simulink model "Tansmissiontest"  (R2024a)
settings: Solver=ode45  StartTime=0.0  StopTime=50  RelTol=1e-3  EnableMultiTasking=on
undefined symbols (not defined in the file): alpha, alpha1, beta, beta1, c, c1, d, gamma, gamma1, k, k1, n, sigma, sigma1
libraries: fl_lib x19, nesl_utility x17, sdl_lib x7, simulink x2
settings Model: Creator=dell  LastModifiedBy=18311
settings SolverCC: AlgebraicLoopSolver=TrustRegion
settings DataIOCC: SaveFormat=StructureWithTime  ReturnWorkspaceOutputs=off
settings OptimizationCC: LifeSpan=inf
settings DebuggingCC: UnconnectedInputMsg=warning  UnconnectedOutputMsg=warning  UnconnectedLineMsg=warning  SFUnexpectedBacktrackingDiag=warning  SFNoUnconditionalDefaultTransitionDiag=warning  SFExecutionAtInitializationDiag=none  ArithmeticOperatorsInVariantConditions=warning
settings HardwareCC: ProdBitPerSizeT=32  ProdBitPerPtrDiffT=32  ProdWordSize=32  ProdHWDeviceType=Specified
settings ModelReferenceCC: EnableRefExpFcnMdlSchedulingChecks=on
settings SFSimCC: SimUseLocalCustomCode=off  CustomCodeUndefinedFunction=UseInterfaceOnly
settings RTWCC: RTWUseLocalCustomCode=off  GPUComputeCapability=3.5  DLArmComputeVersion=19.05
settings CodeAppCC: StateflowObjectComments=on
settings GRTTargetCC: TargetLangStandard=C89/C90 (ANSI)
settings ConfigComp: CovMetricSettings=dw  CovSaveCumulativeToWorkspaceVar=on  CovSaveSingleToWorkspaceVar=on  CovExternalEMLEnable=off
settings SimscapeCC: SimscapeNormalizeSystem=off

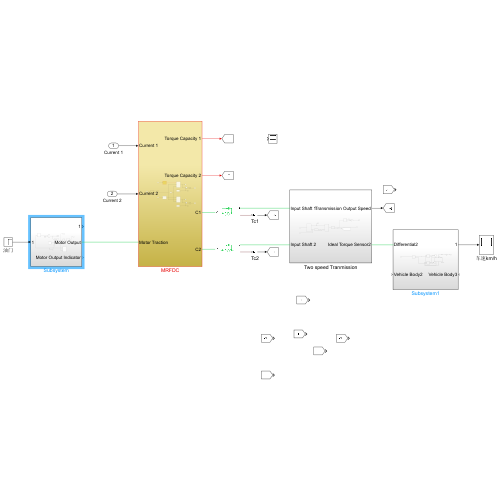
[thumbnail: Simulink's stored preview of the top-level diagram]
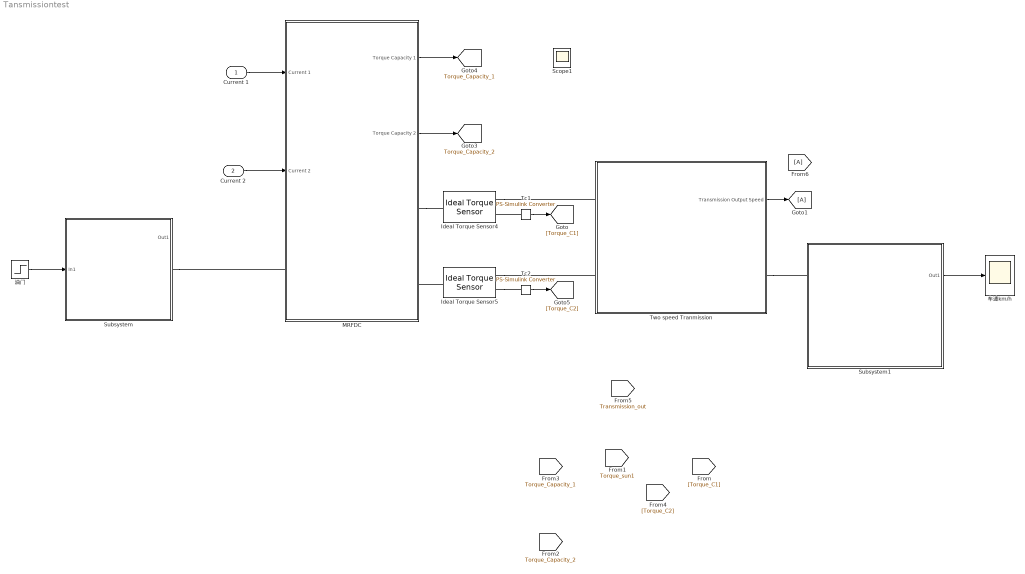
== system Tansmissiontest ==
  Current 1 : Inport
  Current 2 : Inport  Port=2
  From6 : From
  Goto1 : Goto
  Ideal Torque Sensor4 : fl_lib/Mechanical/Mechanical Sensors/Ideal Torque Sensor
  Ideal Torque Sensor5 : fl_lib/Mechanical/Mechanical Sensors/Ideal Torque Sensor
  MRFDC : Subsystem
  Scope1 : Scope
  Subsystem : Subsystem
  Subsystem1 : Subsystem
  Tc1 : nesl_utility/PS-Simulink Converter  PhysicalDomain=network_engine_domain  SubClassName=ps_output  LeftPortType=input  RightPortType=output  PseudoPeriodic=off  Frequencies=[]  VectorFormat=1-D array  Unit=1  AffineConversion=off
  Tc2 : nesl_utility/PS-Simulink Converter  PhysicalDomain=network_engine_domain  SubClassName=ps_output  LeftPortType=input  RightPortType=output  PseudoPeriodic=off  Frequencies=[]  VectorFormat=1-D array  Unit=1  AffineConversion=off
  Two speed Tranmission : Subsystem
  油门 : Step  SampleTime=0
  车速km/h : Scope
  tag scope: Torque_Capacity_1=global, Torque_Capacity_2=global
  wires:
  油门/1 -> Subsystem/1(In1)
  Current 2/1 -> MRFDC/2(Current 2)
  Current 1/1 -> MRFDC/1(Current 1)
  Tc1/1 -> [Torque_C1]
  Tc2/1 -> [Torque_C2]
  MRFDC/1(Torque Capacity 1) -> [Torque_Capacity_1]
  MRFDC/2(Torque Capacity 2) -> [Torque_Capacity_2]
  Subsystem1/1(Out1) -> 车速km/h/1
  Two speed Tranmission/1(Transmission Output Speed) -> Goto1/1
  connections:
  Subsystem/RConn1 -- MRFDC/LConn1
  Ideal Torque Sensor5/LConn1 -- MRFDC/RConn2
  MRFDC/RConn1 -- Ideal Torque Sensor4/LConn1
  Tc1/LConn1 -- Ideal Torque Sensor4/RConn2
  Ideal Torque Sensor5/RConn2 -- Tc2/LConn1
  Ideal Torque Sensor4/RConn1 -- Two speed Tranmission/LConn1
  Ideal Torque Sensor5/RConn1 -- Two speed Tranmission/LConn2
  Two speed Tranmission/RConn1 -- Subsystem1/LConn1

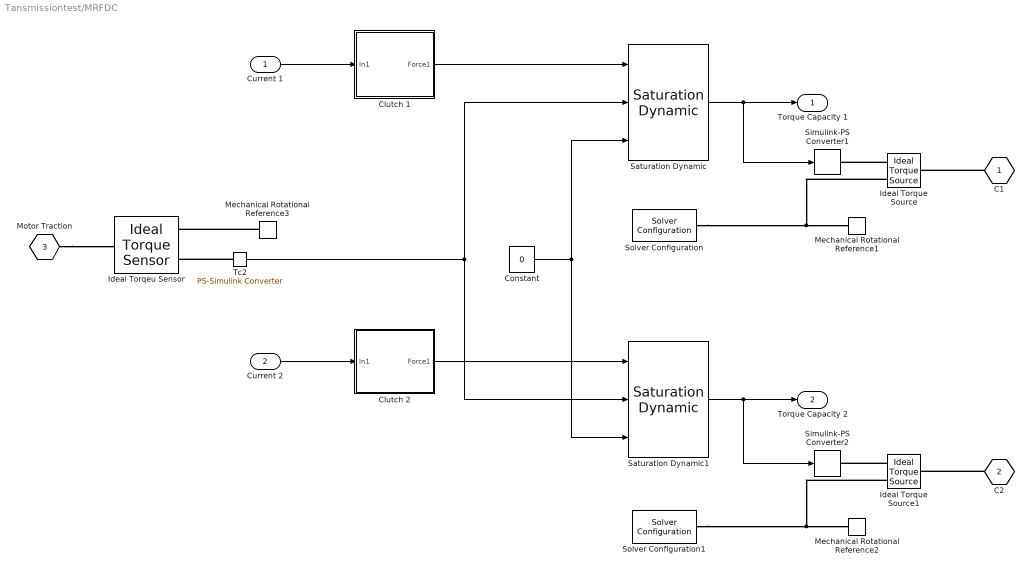
== system Tansmissiontest/MRFDC ==
  Current 1 : Inport
  Current 2 : Inport  Port=2
  Clutch 1 : Subsystem
  Clutch 2 : Subsystem
  Constant : Constant  Value=0
  Ideal Torqeu Sensor : fl_lib/Mechanical/Mechanical Sensors/Ideal Torque Sensor
  Ideal Torque Source : fl_lib/Mechanical/Mechanical Sources/Ideal Torque Source
  Ideal Torque Source1 : fl_lib/Mechanical/Mechanical Sources/Ideal Torque Source
  Mechanical Rotational Reference1 : fl_lib/Mechanical/Rotational Elements/Mechanical Rotational Reference
  Mechanical Rotational Reference2 : fl_lib/Mechanical/Rotational Elements/Mechanical Rotational Reference
  Mechanical Rotational Reference3 : fl_lib/Mechanical/Rotational Elements/Mechanical Rotational Reference
  Saturation Dynamic : simulink/Discontinuities/Saturation Dynamic  OutMin=[]  OutMax=[]  OutDataTypeStr=Inherit: Same as second input  OutDataType=fixdt(1, 16)  OutScaling=2^-10  DoSatur=off
  Saturation Dynamic1 : simulink/Discontinuities/Saturation Dynamic  OutMin=[]  OutMax=[]  OutDataTypeStr=Inherit: Same as second input  OutDataType=fixdt(1, 16)  OutScaling=2^-10  DoSatur=off
  Simulink-PS Converter1 : nesl_utility/Simulink-PS Converter  PhysicalDomain=network_engine_domain  SubClassName=ps_input  LeftPortType=input  RightPortType=output  PseudoPeriodic=off  Frequencies=[]  NoiseDistribution=none  NoiseParameters=[]  Unit=1  AffineConversion=off  FilteringAndDerivatives=zero  SimscapeFilterOrder=1  InputFilterTimeConstant=0.001  UdotUserProvided=1
  Simulink-PS Converter2 : nesl_utility/Simulink-PS Converter  PhysicalDomain=network_engine_domain  SubClassName=ps_input  LeftPortType=input  RightPortType=output  PseudoPeriodic=off  Frequencies=[]  NoiseDistribution=none  NoiseParameters=[]  Unit=1  AffineConversion=off  FilteringAndDerivatives=zero  SimscapeFilterOrder=1  InputFilterTimeConstant=0.001  UdotUserProvided=1
  Solver Configuration : nesl_utility/Solver Configuration  PhysicalDomain=network_engine_domain  SubClassName=solver  LeftPortType=input  RightPortType=generic  Tones=[]  Harmonics=[]  SimulateNoise=off  Profile=off  UseLocalSampling=off  EnableSwitchedLinearOptims=on  FrequencyDomain=off  UseCCode=off  RelTol=0.001  AbsTol=1e-06  MinStep=1e-09  ToWorkspace=off  RevertToSquareIcSolve=off  NumHomotopyIterations=100  PhasorMode=off  PhasorModeNumHarmonics=1  ConsistencySolver=NEWTON_FTOL  IndexReductionMethod=DerivativeReplacement  DoDC=off  ResidualTolerance=1e-09  ConsistencyTolSource=GLOBAL  ConsistencyAbsTol=0.001  ConsistencyRelTol=0.001  ConsistencyTolFactor=0.001  UseLocalSolver=on  LocalSolverChoice=NE_BACKWARD_EULER_ADVANCER  ResolveIndetEquations=on  FunctionEvalNumThread=1  LocalSolverSampleTime=0.001  DoFixedCost=on  MaxNonlinIter=3  MaxModeIter=2  ComputeImpulses=off  ImpulseIterations=2  LinearAlgebra=Sparse  LinearAlgebraNumThread=0  EquationFormulation=NE_TIME_EF  DelaysMemoryBudget=1024  AutomaticFiltering=on  FilteringTimeConstant=0.001  PartitionStorageMethod=AS_NEEDED  PartitionMemoryBudget=1024  PartitionMethod=FAST  MultibodyUseLocalSolver=off  MultibodyLocalSolverChoice=ODE1  MultibodyLocalSolverSampleTime=0.001
  Solver Configuration1 : nesl_utility/Solver Configuration  PhysicalDomain=network_engine_domain  SubClassName=solver  LeftPortType=input  RightPortType=generic  Tones=[]  Harmonics=[]  SimulateNoise=off  Profile=off  UseLocalSampling=off  EnableSwitchedLinearOptims=on  FrequencyDomain=off  UseCCode=off  RelTol=0.001  AbsTol=1e-06  MinStep=1e-09  ToWorkspace=off  RevertToSquareIcSolve=off  NumHomotopyIterations=100  PhasorMode=off  PhasorModeNumHarmonics=1  ConsistencySolver=NEWTON_FTOL  IndexReductionMethod=DerivativeReplacement  DoDC=off  ResidualTolerance=1e-09  ConsistencyTolSource=GLOBAL  ConsistencyAbsTol=0.001  ConsistencyRelTol=0.001  ConsistencyTolFactor=0.001  UseLocalSolver=on  LocalSolverChoice=NE_BACKWARD_EULER_ADVANCER  ResolveIndetEquations=on  FunctionEvalNumThread=1  LocalSolverSampleTime=0.001  DoFixedCost=on  MaxNonlinIter=3  MaxModeIter=2  ComputeImpulses=off  ImpulseIterations=2  LinearAlgebra=Sparse  LinearAlgebraNumThread=0  EquationFormulation=NE_TIME_EF  DelaysMemoryBudget=1024  AutomaticFiltering=on  FilteringTimeConstant=0.001  PartitionStorageMethod=AS_NEEDED  PartitionMemoryBudget=1024  PartitionMethod=FAST  MultibodyUseLocalSolver=off  MultibodyLocalSolverChoice=ODE1  MultibodyLocalSolverSampleTime=0.001
  Tc2 : nesl_utility/PS-Simulink Converter  PhysicalDomain=network_engine_domain  SubClassName=ps_output  LeftPortType=input  RightPortType=output  PseudoPeriodic=off  Frequencies=[]  VectorFormat=1-D array  Unit=1  AffineConversion=off
  C1 : PMIOPort  Side=Right
  C2 : PMIOPort  Port=2  Side=Right
  Motor Traction : PMIOPort  Port=3  Side=Left
  Torque Capacity 1 : Outport
  Torque Capacity 2 : Outport  Port=2
  wires:
  Current 1/1 -> Clutch 1/1(In1)
  Current 2/1 -> Clutch 2/1(In1)
  Clutch 1/1("  Force1") -> Saturation Dynamic/1
  Clutch 2/1("  Force1") -> Saturation Dynamic1/1
  Constant/1 -> Saturation Dynamic/3, Saturation Dynamic1/3
  Saturation Dynamic/1 -> Simulink-PS Converter1/1, Torque Capacity 1/1
  Saturation Dynamic1/1 -> Simulink-PS Converter2/1, Torque Capacity 2/1
  Tc2/1 -> Saturation Dynamic1/2, Saturation Dynamic/2
  connections:
  Ideal Torque Source/RConn1 -- Simulink-PS Converter1/RConn1
  Ideal Torque Source/RConn2 -- Solver Configuration/RConn1 -- Mechanical Rotational Reference1/LConn1
  Ideal Torque Source1/RConn2 -- Solver Configuration1/RConn1 -- Mechanical Rotational Reference2/LConn1
  Ideal Torque Source1/RConn1 -- Simulink-PS Converter2/RConn1
  C1/RConn1 -- Ideal Torque Source/LConn1
  C2/RConn1 -- Ideal Torque Source1/LConn1
  Motor Traction/RConn1 -- Ideal Torqeu Sensor/LConn1
  Tc2/LConn1 -- Ideal Torqeu Sensor/RConn2
  Mechanical Rotational Reference3/LConn1 -- Ideal Torqeu Sensor/RConn1

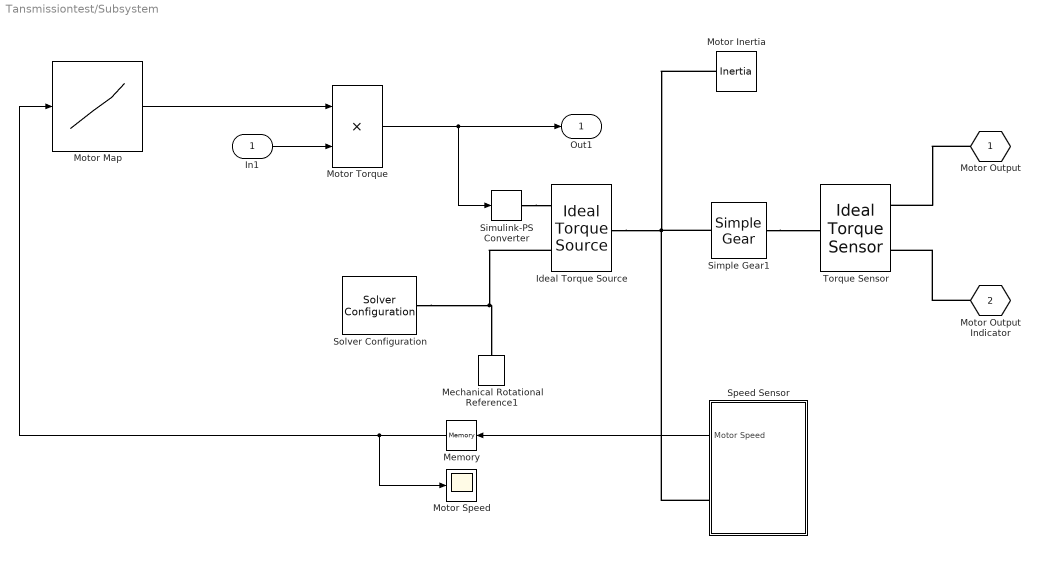
== system Tansmissiontest/Subsystem ==
  In1 : Inport
  Ideal Torque Source : fl_lib/Mechanical/Mechanical Sources/Ideal Torque Source
  Mechanical Rotational Reference1 : fl_lib/Mechanical/Rotational Elements/Mechanical Rotational Reference
  Memory : Memory
  Motor Inertia : fl_lib/Mechanical/Rotational Elements/Inertia  inertia=1 kg*m^2  num_ports=foundation.enum.numPorts2.one  w_specify=off  w_priority=High  w=0 rad/s  w_nominal_specify=off  w_nominal_value=1  w_nominal_unit=rad/s  t_specify=off  t_priority=High  t=0 N*m  t_nominal_specify=off  t_nominal_value=1  t_nominal_unit=N*m
  Motor Map : Lookup_n-D  NumberOfTableDimensions=1  BreakpointsForDimension1="[0 1000 2000 3000 4000 5000 6000 7000  7500]"  Table="[382 382.0000  382.0000  254.6667  191.0000  152.8000  127.3333  109.1429  0]"  InternalRulePriority=Speed  RndMeth=Simplest
  Motor Speed : Scope
  Motor Torque : Product
  Simple Gear1 : sdl_lib/Gears/Simple Gear  ratio=1.6  rotation_direction=3-2*(1)  enable_faults=simscape.enum.onoff.off  efficiency_fault=0.05  fault_angles=pi / 12 rad  friction_model=1  T_noload=0.1 N*m  T_nom=5 N*m  efficiency_nom=0.8  efficiency=0.8  temperature_TLU=[280, 300, 320] K  load_TLU=[1, 5, 10] N*m  efficiency_TLU=[.95, .9, .85]  efficiency_TLU2=[.85, .8, .75; .95, .9, .85; .85, .8, .7]  w_thr=0.01 rad/s  pwr_thr=0.001 W  enable_backlash=false  hardstop_model=simscape.enum.hardstop.smooth  backlash_distance=1e-3 mm  r_base=0.1 m  transition=1e-4 mm  backlash_stiffness=1e7 N/m  backlash_damping=1e6 N*s/m  coeff_rest=0  v_tol=0.001 m/s  f_tol=0 N  mu_visc=[ 0 0 ] N*m/(rad/s)  thermal_mass=50 J/K  temperature_specify=off  temperature_priority=High  temperature=300 K  temperature_nominal_specify=off  temperature_nominal_value=1  temperature_nominal_unit=K  x_backlash_specify=off  x_backlash_priority=None  x_backlash=0 mm  x_backlash_nominal_specify=off  x_backlash_nominal_value=1  x_backlash_nominal_unit=mm  f_hardstop_specify=off  f_hardstop_priority=None  f_hardstop=0 N  f_hardstop_nominal_specify=off  f_hardstop_nominal_value=1  f_hardstop_nominal_unit=N  v_backlash_specify=off  v_backlash_priority=None  v_backlash=0 m/s  v_backlash_nominal_specify=off  v_backlash_nominal_value=1  v_backlash_nominal_unit=m/s
  Simulink-PS Converter : nesl_utility/Simulink-PS Converter  PhysicalDomain=network_engine_domain  SubClassName=ps_input  LeftPortType=input  RightPortType=output  PseudoPeriodic=off  Frequencies=[]  NoiseDistribution=none  NoiseParameters=[]  Unit=1  AffineConversion=off  FilteringAndDerivatives=zero  SimscapeFilterOrder=1  InputFilterTimeConstant=0.001  UdotUserProvided=1
  Solver Configuration : nesl_utility/Solver Configuration  PhysicalDomain=network_engine_domain  SubClassName=solver  LeftPortType=input  RightPortType=generic  Tones=[]  Harmonics=[]  SimulateNoise=off  Profile=off  UseLocalSampling=off  EnableSwitchedLinearOptims=on  FrequencyDomain=off  UseCCode=off  RelTol=0.001  AbsTol=1e-06  MinStep=1e-09  ToWorkspace=off  RevertToSquareIcSolve=off  NumHomotopyIterations=100  PhasorMode=off  PhasorModeNumHarmonics=1  ConsistencySolver=NEWTON_FTOL  IndexReductionMethod=DerivativeReplacement  DoDC=off  ResidualTolerance=1e-09  ConsistencyTolSource=GLOBAL  ConsistencyAbsTol=0.001  ConsistencyRelTol=0.001  ConsistencyTolFactor=0.001  UseLocalSolver=on  LocalSolverChoice=NE_BACKWARD_EULER_ADVANCER  ResolveIndetEquations=on  FunctionEvalNumThread=1  LocalSolverSampleTime=0.001  DoFixedCost=on  MaxNonlinIter=3  MaxModeIter=2  ComputeImpulses=off  ImpulseIterations=2  LinearAlgebra=Sparse  LinearAlgebraNumThread=0  EquationFormulation=NE_TIME_EF  DelaysMemoryBudget=1024  AutomaticFiltering=on  FilteringTimeConstant=0.001  PartitionStorageMethod=AS_NEEDED  PartitionMemoryBudget=1024  PartitionMethod=FAST  MultibodyUseLocalSolver=off  MultibodyLocalSolverChoice=ODE1  MultibodyLocalSolverSampleTime=0.001
  Speed Sensor : Subsystem
  Torque Sensor : fl_lib/Mechanical/Mechanical Sensors/Ideal Torque Sensor
  Motor Output : PMIOPort  Side=Right
  Motor Output Indicator : PMIOPort  Port=2  Side=Right
  Out1 : Outport
  wires:
  Speed Sensor/1(Motor Speed) -> Memory/1
  Motor Torque/1 -> Simulink-PS Converter/1, Out1/1
  Memory/1 -> Motor Map/1, Motor Speed/1
  Motor Map/1 -> Motor Torque/1
  In1/1 -> Motor Torque/2
  connections:
  Ideal Torque Source/RConn2 -- Solver Configuration/RConn1 -- Mechanical Rotational Reference1/LConn1
  Simulink-PS Converter/RConn1 -- Ideal Torque Source/RConn1
  Ideal Torque Source/LConn1 -- Speed Sensor/RConn1 -- Simple Gear1/LConn1 -- Motor Inertia/LConn1
  Simple Gear1/RConn1 -- Torque Sensor/LConn1
  Motor Output/RConn1 -- Torque Sensor/RConn1
  Motor Output Indicator/RConn1 -- Torque Sensor/RConn2

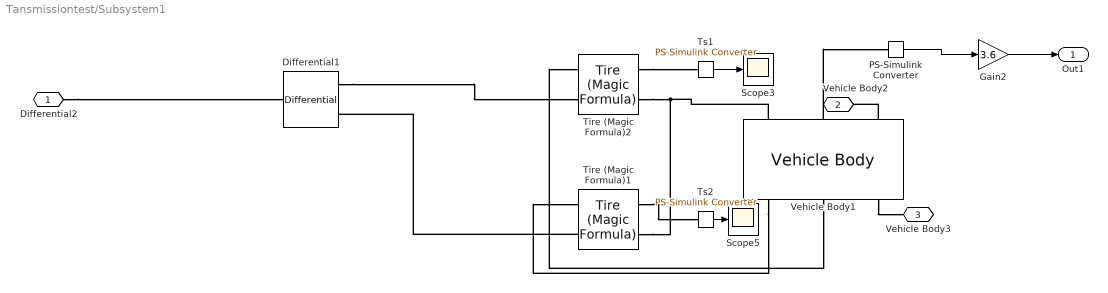
== system Tansmissiontest/Subsystem1 ==
  Differential1 : sdl_lib/Gears/Differential  driveshaft_location=2  cd_ratio=1  friction_model=1  efficiency=[ 0.85 0.92 ]  temperature_TLU=[280, 300, 320] K  efficiency_ss_TLU=[.95, .9, .85]  efficiency_cd_TLU=[.95, .9, .85]  pwr_thr=[.001, .001] W  mu_visc=[ 0 0 ] N*m/(rad/s)  model_inertia=simscape.enum.onoff.off  carrier_inertia=0.001 kg*m^2  planet_inertia=0.001 kg*m^2  thermal_mass=50 J/K  T_init=300 K
  Gain2 : Gain  Gain=3.6
  PS-Simulink Converter : nesl_utility/PS-Simulink Converter  PhysicalDomain=network_engine_domain  SubClassName=ps_output  LeftPortType=input  RightPortType=output  PseudoPeriodic=off  Frequencies=[]  VectorFormat=1-D array  Unit=1  AffineConversion=off
  Scope3 : Scope
  Scope5 : Scope
  Tire (Magic Formula)1 : sdl_lib/Tires & Vehicles/Tire (Magic Formula)  parameterization=1  F_z1=3e+3 N  F_x1=3.5e+3 N  kappa1=10  B_m=10  C_m=1.9  D_m=1  E_m=0.97  fz0=4e+3 N  p_Cx=1.685  p_Dx=[ 1.21 -0.037 ]  p_Ex=[ 0.344 0.095 -0.02 0 ]  p_Kx=[ 21.51 -0.163 0.245 ]  p_Hx=[ -0.002 0.002 ]  p_Vx=[ 0 0 ]  rolling_radius_model=sdl.enum.RollingRadiusParameterization.Constant  r_e=0.3 m  r_0=0.3 m  breff=8.39  dreff=0.26  freff=0.074  q_re0=0.99  q_v1=0.008  longvl=17 m/s  cz=5e5 N/m  model_resistance=1  resistance_model=1  coeff=0.015  p_tire=250e3 Pa  alpha=-0.003  beta=0.97  coeff_a=84e-4  coeff_b=6.2e-4 s/m  coeff_c=1.6e-4 s^2/m^2  p_tire0=240e3 Pa  fz0_resistance=4000 N  vH0=16 m/s  q_Sy=[.0082, 0, .0014, .001, 0, 0, 1.08, -.5]  v_thr=1e-3 m/s  enable_scaling_coefficients=false  lfzO=1  lcx=1  lmux=1  lex=1  lkx=1  lhx=1  lvx=1  lmy=1  model_compliance=0  stiffness=1e+6 N/m  damping=1000 N/(m/s)  model_inertia=1  inertia=1 kg*m^2  initial_velocity=0 rad/s  vxlow=0.1 m/s  v_tr_thr=0.1*(0.1) m/s  kpumin=-1e5  kpumax=1e5
  Tire (Magic Formula)2 : sdl_lib/Tires & Vehicles/Tire (Magic Formula)  parameterization=1  F_z1=3e+3 N  F_x1=3.5e+3 N  kappa1=10  B_m=10  C_m=1.9  D_m=1  E_m=0.97  fz0=4e+3 N  p_Cx=1.685  p_Dx=[ 1.21 -0.037 ]  p_Ex=[ 0.344 0.095 -0.02 0 ]  p_Kx=[ 21.51 -0.163 0.245 ]  p_Hx=[ -0.002 0.002 ]  p_Vx=[ 0 0 ]  rolling_radius_model=sdl.enum.RollingRadiusParameterization.Constant  r_e=0.3 m  r_0=0.3 m  breff=8.39  dreff=0.26  freff=0.074  q_re0=0.99  q_v1=0.008  longvl=17 m/s  cz=5e5 N/m  model_resistance=1  resistance_model=1  coeff=0.015  p_tire=250e3 Pa  alpha=-0.003  beta=0.97  coeff_a=84e-4  coeff_b=6.2e-4 s/m  coeff_c=1.6e-4 s^2/m^2  p_tire0=240e3 Pa  fz0_resistance=4000 N  vH0=16 m/s  q_Sy=[.0082, 0, .0014, .001, 0, 0, 1.08, -.5]  v_thr=1e-3 m/s  enable_scaling_coefficients=false  lfzO=1  lcx=1  lmux=1  lex=1  lkx=1  lhx=1  lvx=1  lmy=1  model_compliance=0  stiffness=1e+6 N/m  damping=1000 N/(m/s)  model_inertia=1  inertia=1 kg*m^2  initial_velocity=0 rad/s  vxlow=0.1 m/s  v_tr_thr=0.1*(0.1) m/s  kpumin=-1e5  kpumax=1e5
  Ts1 : nesl_utility/PS-Simulink Converter  PhysicalDomain=network_engine_domain  SubClassName=ps_output  LeftPortType=input  RightPortType=output  PseudoPeriodic=off  Frequencies=[]  VectorFormat=1-D array  Unit=1  AffineConversion=off
  Ts2 : nesl_utility/PS-Simulink Converter  PhysicalDomain=network_engine_domain  SubClassName=ps_output  LeftPortType=input  RightPortType=output  PseudoPeriodic=off  Frequencies=[]  VectorFormat=1-D array  Unit=1  AffineConversion=off
  Vehicle Body1 : sdl_lib/Tires & Vehicles/Vehicle Body  mass=1500 kg  n_w=2  x_f=1.4 m  x_r=1.6 m  y_c=0.5 m  mass_var=simscape.enum.onoff.off  g=9.81 m/s^2  liftoff_warning=simscape.enum.onoff.off  area=3 m^2  Cd=0.4  rho=1.18 kg/m^3  model_pitch=simscape.enum.onoff.off  inertia=4000 kg*m^2  suspension_model=sdl.enum.linearTLU.linear  k_f=1e4 N/m  b_f=1e4 N/(m/s)  k_r=1e4 N/m  b_r=1e4 N/(m/s)  k_f_TLU=[-2000, -1000, 0, 1000, 2000] N  x_f_TLU=[-.4, -.2, 0, .2, .4] m  b_f_TLU=[-200, -100, 0, 100, 200] N  v_f_TLU=[-4, -2, 0, 2, 4] m/s  k_r_TLU=[-2000, -1000, 0, 1000, 2000] N  x_r_TLU=[-.4, -.2, 0, .2, .4] m  b_r_TLU=[-200, -100, 0, 100, 200] N  v_r_TLU=[-4, -2, 0, 2, 4] m/s  interp_method=simscape.enum.interpolation.linear  extrap_method=simscape.enum.extrapolation.linear  model_hardstop=simscape.enum.onoff.off  upper_bound_f=.25 m  lower_bound_f=-.25 m  stop_k_f=1e6 N/m  stop_b_f=150 N/(m/s)  upper_bound_r=.25 m  lower_bound_r=-.25 m  stop_k_r=1e6 N/m  stop_b_r=150 N/(m/s)  initial_pitch=0 rad  initial_pitch_rate=0 rad/s  v_specify=on  v_priority=High  v=0 m/s  v_nominal_specify=off  v_nominal_value=1  v_nominal_unit=m/s
  Differential2 : PMIOPort  Side=Left
  Vehicle Body2 : PMIOPort  Port=2  Side=Left
  Vehicle Body3 : PMIOPort  Port=3  Side=Right
  Out1 : Outport
  wires:
  Ts2/1 -> Scope5/1
  Gain2/1 -> Out1/1
  PS-Simulink Converter/1 -> Gain2/1
  Ts1/1 -> Scope3/1
  connections:
  Tire (Magic Formula)1/RConn1 -- Ts2/LConn1
  Differential1/RConn2 -- Tire (Magic Formula)2/LConn2
  Vehicle Body1/LConn2 -- PS-Simulink Converter/LConn1
  Vehicle Body1/RConn2 -- Tire (Magic Formula)2/LConn1
  Vehicle Body1/RConn1 -- Tire (Magic Formula)1/LConn1
  Tire (Magic Formula)1/LConn2 -- Differential1/RConn1
  Tire (Magic Formula)2/RConn1 -- Ts1/LConn1
  Tire (Magic Formula)1/RConn2 -- Vehicle Body1/LConn1 -- Tire (Magic Formula)2/RConn2
  Vehicle Body1/RConn3 -- Vehicle Body3/RConn1
  Differential2/RConn1 -- Differential1/LConn1
  Vehicle Body1/LConn3 -- Vehicle Body2/RConn1

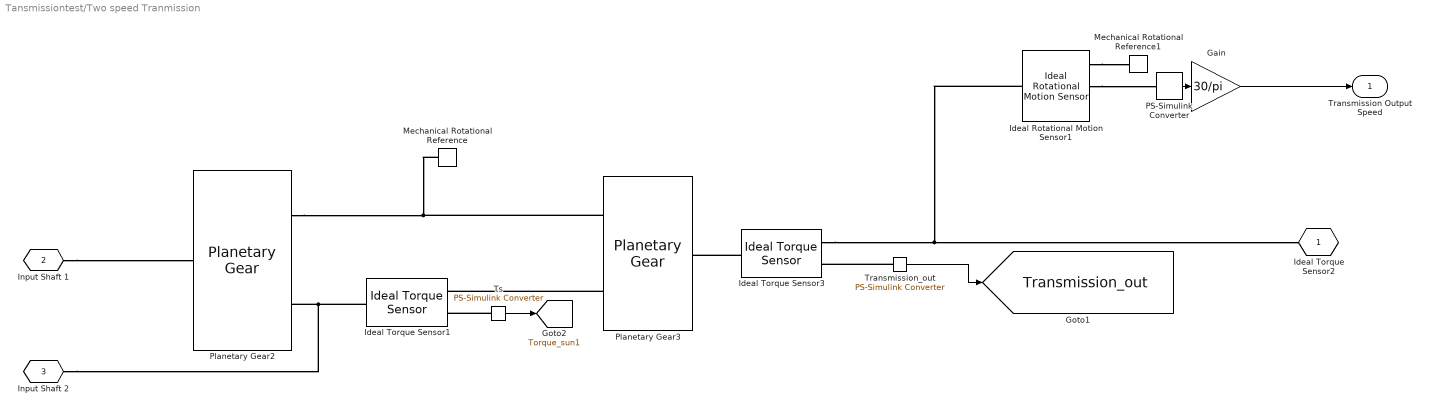
== system Tansmissiontest/Two speed Tranmission ==
  Gain : Gain  Gain=30/pi
  Ideal Rotational Motion Sensor1 : fl_lib/Mechanical/Mechanical Sensors/Ideal Rotational Motion Sensor  reference=foundation.enum.MeasurementReference.difference  acceleration_port=false  velocity_port=true  position_port=true  wrap_angle=simscape.enum.onoff.off  offset=0 rad
  Ideal Torque Sensor1 : fl_lib/Mechanical/Mechanical Sensors/Ideal Torque Sensor
  Ideal Torque Sensor3 : fl_lib/Mechanical/Mechanical Sensors/Ideal Torque Sensor
  Mechanical Rotational Reference : fl_lib/Mechanical/Rotational Elements/Mechanical Rotational Reference
  Mechanical Rotational Reference1 : fl_lib/Mechanical/Rotational Elements/Mechanical Rotational Reference
  PS-Simulink Converter : nesl_utility/PS-Simulink Converter  PhysicalDomain=network_engine_domain  SubClassName=ps_output  LeftPortType=input  RightPortType=output  PseudoPeriodic=off  Frequencies=[]  VectorFormat=1-D array  Unit=1  AffineConversion=off
  Planetary Gear2 : sdl_lib/Gears/Planetary Gear  rs_ratio=1.5  friction_model=1  efficiency=[ 0.96 0.98 ]  temperature_TLU=[280, 300, 320] K  efficiency_sp_TLU=[.95, .9, .85]  efficiency_rp_TLU=[.95, .9, .85]  pwr_thr=[.001, .001] W  mu_visc=[ 0 0 ] N*m/(rad/s)  model_inertia=simscape.enum.onoff.off  planet_inertia=0.001 kg*m^2  thermal_mass=50 J/K  T_init=300 K
  Planetary Gear3 : sdl_lib/Gears/Planetary Gear  rs_ratio=3  friction_model=1  efficiency=[ 0.96 0.98 ]  temperature_TLU=[280, 300, 320] K  efficiency_sp_TLU=[.95, .9, .85]  efficiency_rp_TLU=[.95, .9, .85]  pwr_thr=[.001, .001] W  mu_visc=[ 0 0 ] N*m/(rad/s)  model_inertia=simscape.enum.onoff.off  planet_inertia=0.001 kg*m^2  thermal_mass=50 J/K  T_init=300 K
  Transmission_out : nesl_utility/PS-Simulink Converter  PhysicalDomain=network_engine_domain  SubClassName=ps_output  LeftPortType=input  RightPortType=output  PseudoPeriodic=off  Frequencies=[]  VectorFormat=1-D array  Unit=1  AffineConversion=off
  Ts : nesl_utility/PS-Simulink Converter  PhysicalDomain=network_engine_domain  SubClassName=ps_output  LeftPortType=input  RightPortType=output  PseudoPeriodic=off  Frequencies=[]  VectorFormat=1-D array  Unit=1  AffineConversion=off
  Ideal Torque Sensor2 : PMIOPort  Side=Right
  Input Shaft 1 : PMIOPort  Port=2  Side=Left
  Input Shaft 2 : PMIOPort  Port=3  Side=Left
  Transmission Output Speed : Outport
  tag scope: Torque_sun1=global, Transmission_out=global
  wires:
  Ts/1 -> [Torque_sun1]
  Transmission_out/1 -> [Transmission_out]
  PS-Simulink Converter/1 -> Gain/1
  Gain/1 -> Transmission Output Speed/1
  connections:
  Ts/LConn1 -- Ideal Torque Sensor1/RConn2
  Ideal Torque Sensor1/LConn1 -- Input Shaft 2/RConn1 -- Planetary Gear2/RConn2
  Planetary Gear3/RConn2 -- Ideal Torque Sensor1/RConn1
  Mechanical Rotational Reference/LConn1 -- Planetary Gear3/RConn1 -- Planetary Gear2/RConn1
  Ideal Torque Sensor3/LConn1 -- Planetary Gear3/LConn1
  Transmission_out/LConn1 -- Ideal Torque Sensor3/RConn2
  Ideal Torque Sensor3/RConn1 -- Ideal Rotational Motion Sensor1/LConn1 -- Ideal Torque Sensor2/RConn1
  Input Shaft 1/RConn1 -- Planetary Gear2/LConn1
  Ideal Rotational Motion Sensor1/RConn1 -- Mechanical Rotational Reference1/LConn1
  Ideal Rotational Motion Sensor1/RConn2 -- PS-Simulink Converter/LConn1

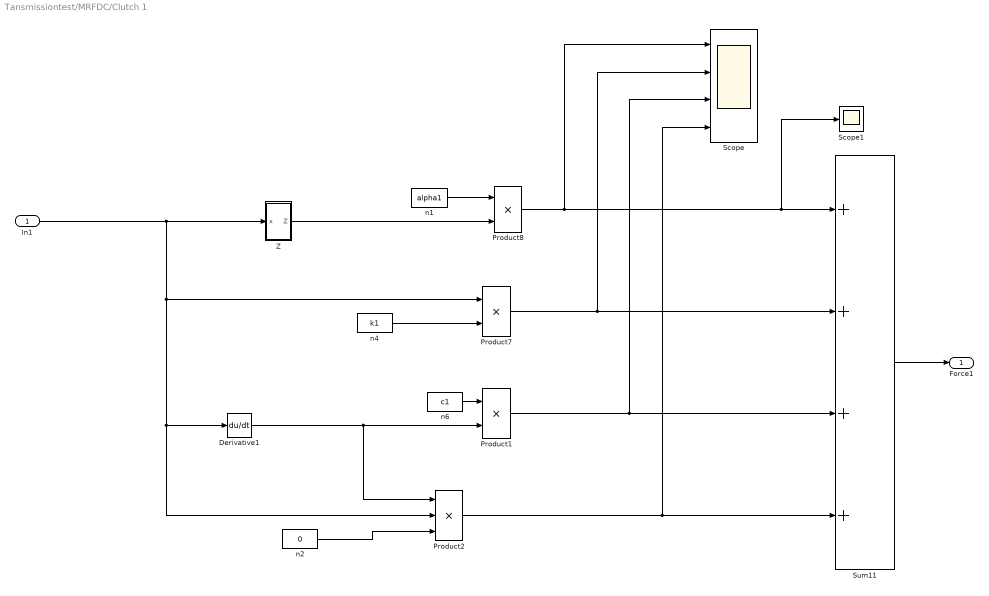
== system Tansmissiontest/MRFDC/Clutch 1 ==
  In1 : Inport
  Derivative1 : Derivative
  Product1 : Product  InputSameDT=on  SaturateOnIntegerOverflow=on  OutDataTypeStr=Inherit: Same as first input
  Product2 : Product  Inputs=3  InputSameDT=on  SaturateOnIntegerOverflow=on  OutDataTypeStr=Inherit: Same as first input
  Product7 : Product  InputSameDT=on  SaturateOnIntegerOverflow=on  OutDataTypeStr=Inherit: Same as first input
  Product8 : Product  InputSameDT=on  SaturateOnIntegerOverflow=on  OutDataTypeStr=Inherit: Same as first input
  Scope : Scope  NumInputPorts=4
  Scope1 : Scope
  Sum11 : Sum  Inputs=++++  InputSameDT=on  SaturateOnIntegerOverflow=on  OutDataTypeStr=Inherit: Same as first input
  Z : Subsystem
  n1 : Constant  Value=alpha1
  n2 : Constant  Value=0
  n4 : Constant  Value=k1
  n6 : Constant  Value=c1
  "  Force1" : Outport
  wires:
  Z/1(Z) -> Product8/2
  Product8/1 -> Scope/1, Scope1/1, Sum11/1
  n1/1 -> Product8/1
  Product7/1 -> Scope/2, Sum11/2
  n4/1 -> Product7/2
  Sum11/1 -> "  Force1"/1
  In1/1 -> Z/1(x), Product7/1, Product2/2, Derivative1/1
  Product1/1 -> Scope/3, Sum11/3
  Derivative1/1 -> Product2/1, Product1/2
  n6/1 -> Product1/1
  n2/1 -> Product2/3
  Product2/1 -> Scope/4, Sum11/4

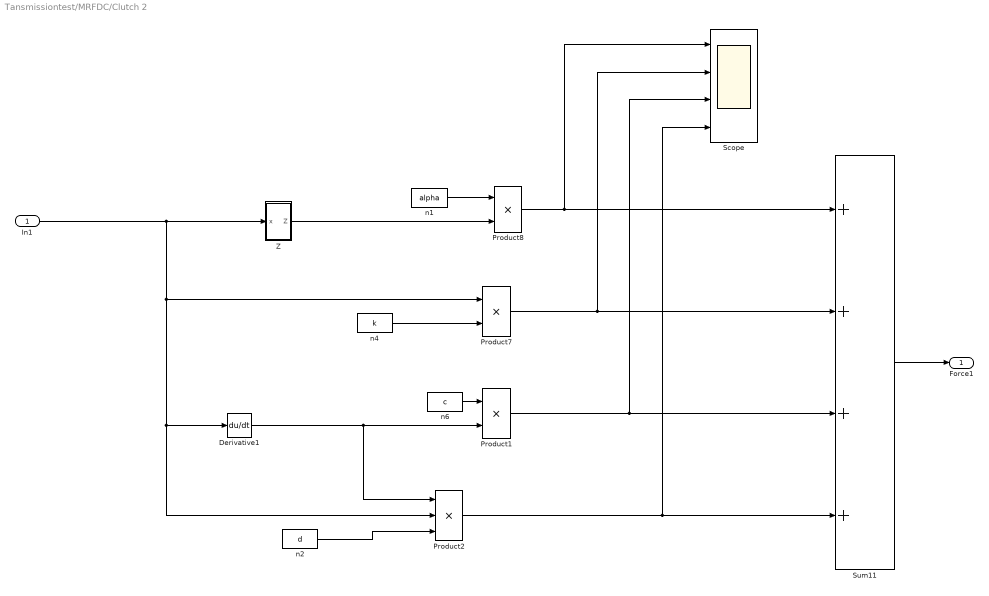
== system Tansmissiontest/MRFDC/Clutch 2 ==
  In1 : Inport
  Derivative1 : Derivative
  Product1 : Product  InputSameDT=on  SaturateOnIntegerOverflow=on  OutDataTypeStr=Inherit: Same as first input
  Product2 : Product  Inputs=3  InputSameDT=on  SaturateOnIntegerOverflow=on  OutDataTypeStr=Inherit: Same as first input
  Product7 : Product  InputSameDT=on  SaturateOnIntegerOverflow=on  OutDataTypeStr=Inherit: Same as first input
  Product8 : Product  InputSameDT=on  SaturateOnIntegerOverflow=on  OutDataTypeStr=Inherit: Same as first input
  Scope : Scope  NumInputPorts=4
  Sum11 : Sum  Inputs=++++  InputSameDT=on  SaturateOnIntegerOverflow=on  OutDataTypeStr=Inherit: Same as first input
  Z : Subsystem
  n1 : Constant  Value=alpha
  n2 : Constant  Value=d
  n4 : Constant  Value=k
  n6 : Constant  Value=c
  "  Force1" : Outport
  wires:
  Product2/1 -> Sum11/4, Scope/4
  n2/1 -> Product2/3
  n6/1 -> Product1/1
  Derivative1/1 -> Product1/2, Product2/1
  Product1/1 -> Sum11/3, Scope/3
  In1/1 -> Derivative1/1, Product2/2, Product7/1, Z/1(x)
  Sum11/1 -> "  Force1"/1
  n4/1 -> Product7/2
  Product7/1 -> Sum11/2, Scope/2
  n1/1 -> Product8/1
  Product8/1 -> Sum11/1, Scope/1
  Z/1(Z) -> Product8/2

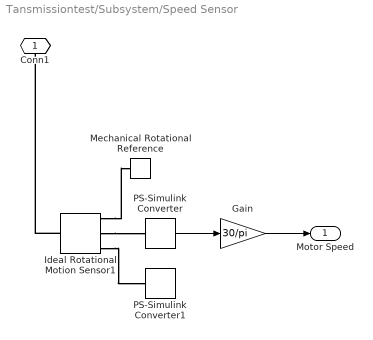
== system Tansmissiontest/Subsystem/Speed Sensor ==
  Gain : Gain  Gain=30/pi
  Ideal Rotational Motion Sensor1 : fl_lib/Mechanical/Mechanical Sensors/Ideal Rotational Motion Sensor  reference=foundation.enum.MeasurementReference.difference  acceleration_port=false  velocity_port=true  position_port=true  wrap_angle=simscape.enum.onoff.off  offset=0 rad
  Mechanical Rotational Reference : fl_lib/Mechanical/Rotational Elements/Mechanical Rotational Reference
  PS-Simulink Converter : nesl_utility/PS-Simulink Converter  PhysicalDomain=network_engine_domain  SubClassName=ps_output  LeftPortType=input  RightPortType=output  PseudoPeriodic=off  Frequencies=[]  VectorFormat=1-D array  Unit=1  AffineConversion=off
  PS-Simulink Converter1 : nesl_utility/PS-Simulink Converter  PhysicalDomain=network_engine_domain  SubClassName=ps_output  LeftPortType=input  RightPortType=output  PseudoPeriodic=off  Frequencies=[]  VectorFormat=1-D array  Unit=1  AffineConversion=off
  Conn1 : PMIOPort  Side=Right
  Motor Speed : Outport
  wires:
  PS-Simulink Converter/1 -> Gain/1
  Gain/1 -> Motor Speed/1
  connections:
  Ideal Rotational Motion Sensor1/RConn1 -- Mechanical Rotational Reference/LConn1
  Ideal Rotational Motion Sensor1/RConn3 -- PS-Simulink Converter1/LConn1
  Ideal Rotational Motion Sensor1/LConn1 -- Conn1/RConn1
  Ideal Rotational Motion Sensor1/RConn2 -- PS-Simulink Converter/LConn1

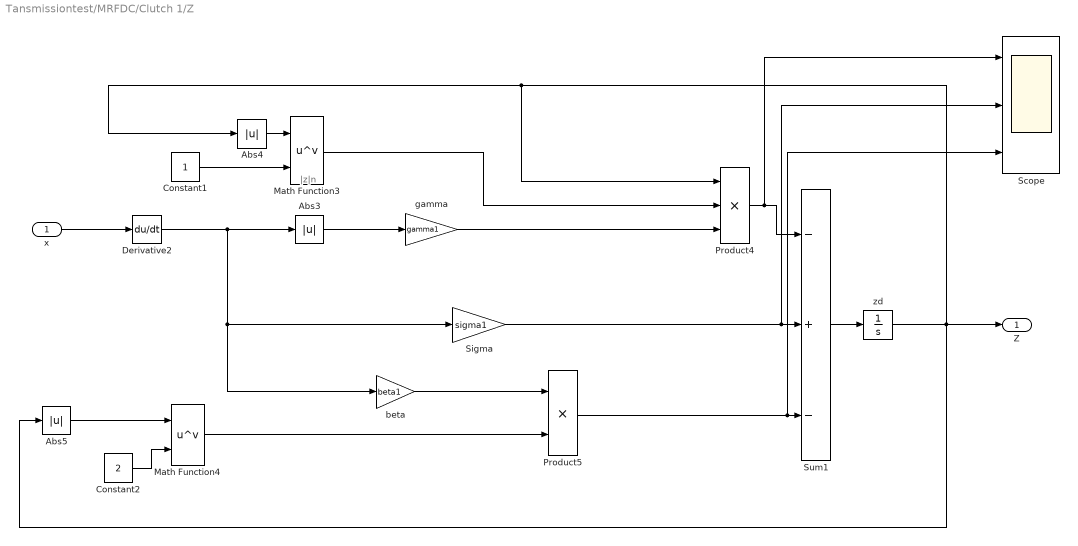
== system Tansmissiontest/MRFDC/Clutch 1/Z ==
  note: |z|n
  x : Inport
  Abs3 : Abs  ZeroCross=off
  Abs4 : Abs  ZeroCross=off
  Abs5 : Abs  ZeroCross=off
  Constant1 : Constant
  Constant2 : Constant  Value=2
  Derivative2 : Derivative
  Math Function3 : Math  Operator=pow  SignedPower=on  OutputSignalType=real
  Math Function4 : Math  Operator=pow  SignedPower=on  OutputSignalType=real
  Product4 : Product  Inputs=3  InputSameDT=on  SaturateOnIntegerOverflow=on  OutDataTypeStr=Inherit: Same as first input
  Product5 : Product  InputSameDT=on  SaturateOnIntegerOverflow=on  OutDataTypeStr=Inherit: Same as first input
  Scope : Scope  NumInputPorts=3
  Sigma : Gain  Gain=sigma1  SaturateOnIntegerOverflow=on  OutDataTypeStr=Inherit: Same as input  ParamDataTypeStr=Inherit: Same as input
  Sum1 : Sum  Inputs=-+-  InputSameDT=on  SaturateOnIntegerOverflow=on  OutDataTypeStr=Inherit: Same as first input
  beta : Gain  Gain=beta1  SaturateOnIntegerOverflow=on  OutDataTypeStr=Inherit: Same as input  ParamDataTypeStr=Inherit: Same as input
  gamma : Gain  Gain=gamma1  SaturateOnIntegerOverflow=on  OutDataTypeStr=Inherit: Same as input  ParamDataTypeStr=Inherit: Same as input
  zd : Integrator  LimitOutput=on  UpperSaturationLimit=1000  LowerSaturationLimit=-1000
  Z : Outport  VectorParamsAs1DForOutWhenUnconnected=off
  wires:
  Abs4/1 -> Math Function3/1
  Math Function3/1 -> Product4/2
  x/1 -> Derivative2/1
  Product5/1 -> Scope/3, Sum1/3
  zd/1 -> Abs5/1, Z/1, Product4/1, Abs4/1
  Derivative2/1 -> Sigma/1, beta/1, Abs3/1
  Math Function4/1 -> Product5/2
  Abs3/1 -> gamma/1
  Abs5/1 -> Math Function4/1
  Sigma/1 -> Scope/2, Sum1/2
  gamma/1 -> Product4/3
  Product4/1 -> Scope/1, Sum1/1
  beta/1 -> Product5/1
  Sum1/1 -> zd/1
  Constant1/1 -> Math Function3/2
  Constant2/1 -> Math Function4/2

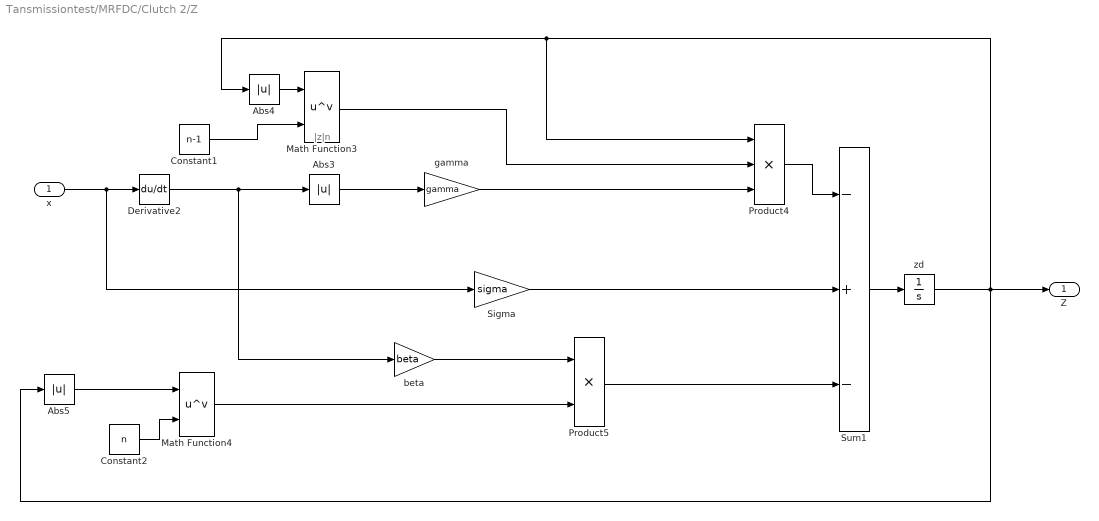
== system Tansmissiontest/MRFDC/Clutch 2/Z ==
  note: |z|n
  x : Inport
  Abs3 : Abs  ZeroCross=off
  Abs4 : Abs  ZeroCross=off
  Abs5 : Abs  ZeroCross=off
  Constant1 : Constant  Value=n-1
  Constant2 : Constant  Value=n
  Derivative2 : Derivative
  Math Function3 : Math  Operator=pow  SignedPower=on  OutputSignalType=real
  Math Function4 : Math  Operator=pow  SignedPower=on  OutputSignalType=real
  Product4 : Product  Inputs=3  InputSameDT=on  SaturateOnIntegerOverflow=on  OutDataTypeStr=Inherit: Same as first input
  Product5 : Product  InputSameDT=on  SaturateOnIntegerOverflow=on  OutDataTypeStr=Inherit: Same as first input
  Sigma : Gain  Gain=sigma  SaturateOnIntegerOverflow=on  OutDataTypeStr=Inherit: Same as input  ParamDataTypeStr=Inherit: Same as input
  Sum1 : Sum  Inputs=-+-  InputSameDT=on  SaturateOnIntegerOverflow=on  OutDataTypeStr=Inherit: Same as first input
  beta : Gain  Gain=beta  SaturateOnIntegerOverflow=on  OutDataTypeStr=Inherit: Same as input  ParamDataTypeStr=Inherit: Same as input
  gamma : Gain  Gain=gamma  SaturateOnIntegerOverflow=on  OutDataTypeStr=Inherit: Same as input  ParamDataTypeStr=Inherit: Same as input
  zd : Integrator  LimitOutput=on  UpperSaturationLimit=1000  LowerSaturationLimit=-1000
  Z : Outport  VectorParamsAs1DForOutWhenUnconnected=off
  wires:
  Constant2/1 -> Math Function4/2
  Constant1/1 -> Math Function3/2
  Sum1/1 -> zd/1
  beta/1 -> Product5/1
  Product4/1 -> Sum1/1
  gamma/1 -> Product4/3
  Sigma/1 -> Sum1/2
  Abs5/1 -> Math Function4/1
  Abs3/1 -> gamma/1
  Math Function4/1 -> Product5/2
  Derivative2/1 -> Abs3/1, beta/1
  zd/1 -> Abs4/1, Product4/1, Z/1, Abs5/1
  Product5/1 -> Sum1/3
  x/1 -> Derivative2/1, Sigma/1
  Math Function3/1 -> Product4/2
  Abs4/1 -> Math Function3/1
